simulink model "Modelado_Dron_cuadricoptero_v3"  (R2023a)
settings: Solver=VariableStepAuto  StartTime=0.0  StopTime=10  RelTol=1e-3
libraries: slpidlib x3, sim3dlib x1, uavsim3dlib x1
settings Model: Creator=enzog  LastModifiedBy=enzog

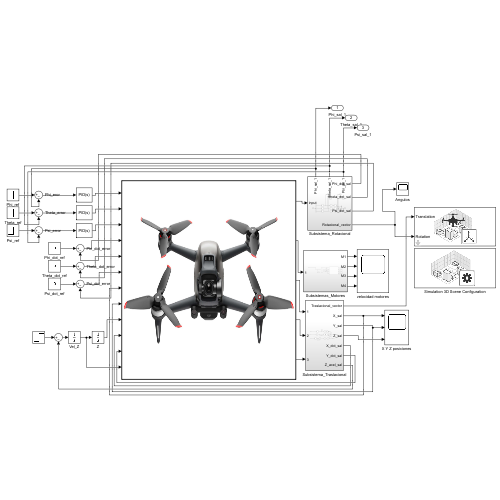
[thumbnail: Simulink's stored preview of the top-level diagram]
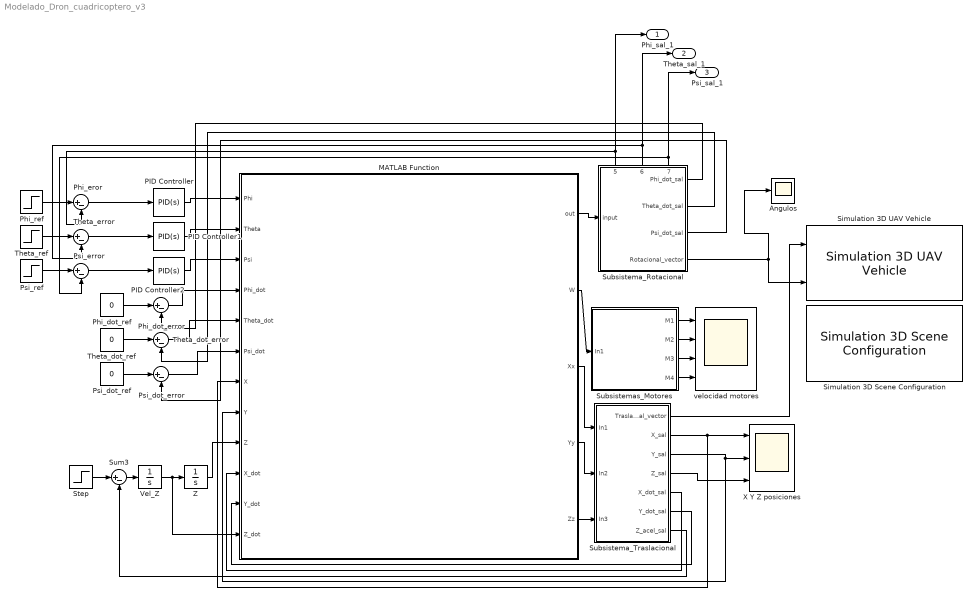
== system Modelado_Dron_cuadricoptero_v3 ==
  Angulos : Scope
  MATLAB Function : MATLAB Function  TreatAsAtomicUnit=on
  PID Controller : slpidlib/PID Controller  Controller=PID  Form=Parallel  TimeDomain=Continuous-time  UseExternalTs=off  SampleTime=-1  IntegratorMethod=Forward Euler  FilterMethod=Forward Euler  ControllerParametersSource=internal  P=150  I=700  UseKiTs=off  D=57  N=100  UseFilter=on  TunerSelectOption=Transfer Function Based (PID Tuner App)  InitialConditionSource=internal  InitialConditionForIntegrator=0  InitialConditionForFilter=0  DifferentiatorICPrevScaledInput=0  ExternalReset=none  TrackingMode=off  Kt=1  LimitOutput=off  SatLimitsSource=internal  UpperSaturationLimit=inf  LowerSaturationLimit=-inf  LinearizeAsGain=on  AntiWindupMode=none  Kb=1  LimitIntegrator=off  UpperIntegratorSaturationLimit=inf  LowerIntegratorSaturationLimit=-inf  POutMin=[]  POutMax=[]  IOutMin=[]  IOutMax=[]  DOutMin=[]  DOutMax=[]  NOutMin=[]  NOutMax=[]  SumOutMin=[]  SumOutMax=[]  SaturationOutMin=[]  SaturationOutMax=[]  PParamMin=[]  PParamMax=[]  IParamMin=[]  IParamMax=[]  DParamMin=[]  DParamMax=[]  NParamMin=[]  NParamMax=[]  KbParamMin=[]  KbParamMax=[]  KtParamMin=[]  KtParamMax=[]  KbOutMin=[]  KbOutMax=[]  KtOutMin=[]  KtOutMax=[]  IntegratorOutMin=[]  IntegratorOutMax=[]  FilterOutMin=[]  FilterOutMax=[]  SumI1OutMin=[]  SumI1OutMax=[]  SumI2OutMin=[]  SumI2OutMax=[]  SumI3OutMin=[]  SumI3OutMax=[]  SumI4OutMin=[]  SumI4OutMax=[]  SumDOutMin=[]  SumDOutMax=[]  DifferentiatorOutMin=[]  DifferentiatorOutMax=[]  FilterDiffOutCoefMin=[]  FilterDiffOutCoefMax=[]  ReciprocalOutMin=[]  ReciprocalOutMax=[]  SumDenOutMin=[]  SumDenOutMax=[]  SumNumOutMin=[]  SumNumOutMax=[]  DivideOutMin=[]  DivideOutMax=[]  UdiffTsProdOutMin=[]  UdiffTsProdOutMax=[]  NTsProdOutMin=[]  NTsProdOutMax=[]  UintegralTsProdOutMin=[]  UintegralTsProdOutMax=[]  UngainTsProdOutMin=[]  UngainTsProdOutMax=[]  ClampingZeroOutDataTypeStr=Inherit: Inherit via back propagation  ClampingZeroOutMin=[]  ClampingZeroOutMax=[]  FilterDenConstantOutDataTypeStr=Inherit: Inherit via back propagation  FilterDenConstantOutMin=[]  FilterDenConstantOutMax=[]  PCopyOutDataTypeStr=Inherit: Inherit via back propagation  PCopyOutMin=[]  PCopyOutMax=[]  NCopyOutDataTypeStr=Inherit: Inherit via back propagation  NCopyOutMin=[]  NCopyOutMax=[]  IntegratorContinuousStateAttributes=''  IntegratorStateMustResolveToSignalObject=off  IntegratorRTWStateStorageClass=Auto  FilterContinuousStateAttributes=''  FilterStateMustResolveToSignalObject=off  FilterRTWStateStorageClass=Auto  ParallelPVariant=InternalParameters  IdealPVariant=Disabled  IVariant=InternalParameters  DVariant=InternalParameters  IntegratorVariant=Continuous  SatVariant=Disabled  AWVariant=Passthrough  PCopyVariant=Disabled  TRVariant=Disabled  FdbkBlocksVariant=Forward  IdealPFdbkVariant=Disabled  SatFdbkVariant=Disabled  DerivativeFilterVariant=ContFilter  NVariant=InternalParameters  NCopyVariant=Disabled  FilterICVariant=InternalICsFilter  IntegratorICVariant=InternalICs  ExternalResetVariant=Disabled  TRSumVariant=Passthrough  SumFdbkVariant=Disabled  SumVariant=Sum_PID  TsampFilterVariant=InternalTs  TsampNgainVariant=Passthrough  TsampIntegralVariant=Disabled_SignalSpec  ExternalSaturationOutDataTypeStr=Inherit: Same as second input
  PID Controller1 : slpidlib/PID Controller  Controller=PID  Form=Parallel  TimeDomain=Continuous-time  UseExternalTs=off  SampleTime=-1  IntegratorMethod=Forward Euler  FilterMethod=Forward Euler  ControllerParametersSource=internal  P=400  I=8.5  UseKiTs=off  D=25  N=100  UseFilter=on  TunerSelectOption=Transfer Function Based (PID Tuner App)  InitialConditionSource=internal  InitialConditionForIntegrator=0  InitialConditionForFilter=0  DifferentiatorICPrevScaledInput=0  ExternalReset=none  TrackingMode=off  Kt=1  LimitOutput=off  SatLimitsSource=internal  UpperSaturationLimit=inf  LowerSaturationLimit=-inf  LinearizeAsGain=on  AntiWindupMode=none  Kb=1  LimitIntegrator=off  UpperIntegratorSaturationLimit=inf  LowerIntegratorSaturationLimit=-inf  POutMin=[]  POutMax=[]  IOutMin=[]  IOutMax=[]  DOutMin=[]  DOutMax=[]  NOutMin=[]  NOutMax=[]  SumOutMin=[]  SumOutMax=[]  SaturationOutMin=[]  SaturationOutMax=[]  PParamMin=[]  PParamMax=[]  IParamMin=[]  IParamMax=[]  DParamMin=[]  DParamMax=[]  NParamMin=[]  NParamMax=[]  KbParamMin=[]  KbParamMax=[]  KtParamMin=[]  KtParamMax=[]  KbOutMin=[]  KbOutMax=[]  KtOutMin=[]  KtOutMax=[]  IntegratorOutMin=[]  IntegratorOutMax=[]  FilterOutMin=[]  FilterOutMax=[]  SumI1OutMin=[]  SumI1OutMax=[]  SumI2OutMin=[]  SumI2OutMax=[]  SumI3OutMin=[]  SumI3OutMax=[]  SumI4OutMin=[]  SumI4OutMax=[]  SumDOutMin=[]  SumDOutMax=[]  DifferentiatorOutMin=[]  DifferentiatorOutMax=[]  FilterDiffOutCoefMin=[]  FilterDiffOutCoefMax=[]  ReciprocalOutMin=[]  ReciprocalOutMax=[]  SumDenOutMin=[]  SumDenOutMax=[]  SumNumOutMin=[]  SumNumOutMax=[]  DivideOutMin=[]  DivideOutMax=[]  UdiffTsProdOutMin=[]  UdiffTsProdOutMax=[]  NTsProdOutMin=[]  NTsProdOutMax=[]  UintegralTsProdOutMin=[]  UintegralTsProdOutMax=[]  UngainTsProdOutMin=[]  UngainTsProdOutMax=[]  ClampingZeroOutDataTypeStr=Inherit: Inherit via back propagation  ClampingZeroOutMin=[]  ClampingZeroOutMax=[]  FilterDenConstantOutDataTypeStr=Inherit: Inherit via back propagation  FilterDenConstantOutMin=[]  FilterDenConstantOutMax=[]  PCopyOutDataTypeStr=Inherit: Inherit via back propagation  PCopyOutMin=[]  PCopyOutMax=[]  NCopyOutDataTypeStr=Inherit: Inherit via back propagation  NCopyOutMin=[]  NCopyOutMax=[]  IntegratorContinuousStateAttributes=''  IntegratorStateMustResolveToSignalObject=off  IntegratorRTWStateStorageClass=Auto  FilterContinuousStateAttributes=''  FilterStateMustResolveToSignalObject=off  FilterRTWStateStorageClass=Auto  ParallelPVariant=InternalParameters  IdealPVariant=Disabled  IVariant=InternalParameters  DVariant=InternalParameters  IntegratorVariant=Continuous  SatVariant=Disabled  AWVariant=Passthrough  PCopyVariant=Disabled  TRVariant=Disabled  FdbkBlocksVariant=Forward  IdealPFdbkVariant=Disabled  SatFdbkVariant=Disabled  DerivativeFilterVariant=ContFilter  NVariant=InternalParameters  NCopyVariant=Disabled  FilterICVariant=InternalICsFilter  IntegratorICVariant=InternalICs  ExternalResetVariant=Disabled  TRSumVariant=Passthrough  SumFdbkVariant=Disabled  SumVariant=Sum_PID  TsampFilterVariant=InternalTs  TsampNgainVariant=Passthrough  TsampIntegralVariant=Disabled_SignalSpec  ExternalSaturationOutDataTypeStr=Inherit: Same as second input
  PID Controller2 : slpidlib/PID Controller  Controller=PID  Form=Parallel  TimeDomain=Continuous-time  UseExternalTs=off  SampleTime=-1  IntegratorMethod=Forward Euler  FilterMethod=Forward Euler  ControllerParametersSource=internal  P=50  I=5.5  UseKiTs=off  D=10  N=100  UseFilter=on  TunerSelectOption=Transfer Function Based (PID Tuner App)  InitialConditionSource=internal  InitialConditionForIntegrator=0  InitialConditionForFilter=0  DifferentiatorICPrevScaledInput=0  ExternalReset=none  TrackingMode=off  Kt=1  LimitOutput=off  SatLimitsSource=internal  UpperSaturationLimit=inf  LowerSaturationLimit=-inf  LinearizeAsGain=on  AntiWindupMode=none  Kb=1  LimitIntegrator=off  UpperIntegratorSaturationLimit=inf  LowerIntegratorSaturationLimit=-inf  POutMin=[]  POutMax=[]  IOutMin=[]  IOutMax=[]  DOutMin=[]  DOutMax=[]  NOutMin=[]  NOutMax=[]  SumOutMin=[]  SumOutMax=[]  SaturationOutMin=[]  SaturationOutMax=[]  PParamMin=[]  PParamMax=[]  IParamMin=[]  IParamMax=[]  DParamMin=[]  DParamMax=[]  NParamMin=[]  NParamMax=[]  KbParamMin=[]  KbParamMax=[]  KtParamMin=[]  KtParamMax=[]  KbOutMin=[]  KbOutMax=[]  KtOutMin=[]  KtOutMax=[]  IntegratorOutMin=[]  IntegratorOutMax=[]  FilterOutMin=[]  FilterOutMax=[]  SumI1OutMin=[]  SumI1OutMax=[]  SumI2OutMin=[]  SumI2OutMax=[]  SumI3OutMin=[]  SumI3OutMax=[]  SumI4OutMin=[]  SumI4OutMax=[]  SumDOutMin=[]  SumDOutMax=[]  DifferentiatorOutMin=[]  DifferentiatorOutMax=[]  FilterDiffOutCoefMin=[]  FilterDiffOutCoefMax=[]  ReciprocalOutMin=[]  ReciprocalOutMax=[]  SumDenOutMin=[]  SumDenOutMax=[]  SumNumOutMin=[]  SumNumOutMax=[]  DivideOutMin=[]  DivideOutMax=[]  UdiffTsProdOutMin=[]  UdiffTsProdOutMax=[]  NTsProdOutMin=[]  NTsProdOutMax=[]  UintegralTsProdOutMin=[]  UintegralTsProdOutMax=[]  UngainTsProdOutMin=[]  UngainTsProdOutMax=[]  ClampingZeroOutDataTypeStr=Inherit: Inherit via back propagation  ClampingZeroOutMin=[]  ClampingZeroOutMax=[]  FilterDenConstantOutDataTypeStr=Inherit: Inherit via back propagation  FilterDenConstantOutMin=[]  FilterDenConstantOutMax=[]  PCopyOutDataTypeStr=Inherit: Inherit via back propagation  PCopyOutMin=[]  PCopyOutMax=[]  NCopyOutDataTypeStr=Inherit: Inherit via back propagation  NCopyOutMin=[]  NCopyOutMax=[]  IntegratorContinuousStateAttributes=''  IntegratorStateMustResolveToSignalObject=off  IntegratorRTWStateStorageClass=Auto  FilterContinuousStateAttributes=''  FilterStateMustResolveToSignalObject=off  FilterRTWStateStorageClass=Auto  ParallelPVariant=InternalParameters  IdealPVariant=Disabled  IVariant=InternalParameters  DVariant=InternalParameters  IntegratorVariant=Continuous  SatVariant=Disabled  AWVariant=Passthrough  PCopyVariant=Disabled  TRVariant=Disabled  FdbkBlocksVariant=Forward  IdealPFdbkVariant=Disabled  SatFdbkVariant=Disabled  DerivativeFilterVariant=ContFilter  NVariant=InternalParameters  NCopyVariant=Disabled  FilterICVariant=InternalICsFilter  IntegratorICVariant=InternalICs  ExternalResetVariant=Disabled  TRSumVariant=Passthrough  SumFdbkVariant=Disabled  SumVariant=Sum_PID  TsampFilterVariant=InternalTs  TsampNgainVariant=Passthrough  TsampIntegralVariant=Disabled_SignalSpec  ExternalSaturationOutDataTypeStr=Inherit: Same as second input
  Phi_dot_error : Sum  Inputs=|+-
  Phi_dot_ref : Constant  Value=0
  Phi_eror : Sum  Inputs=|+-
  Phi_ref : Step  Time=4  After=0.3  SampleTime=0
  Psi_dot_error : Sum  Inputs=|+-
  Psi_dot_ref : Constant  Value=0
  Psi_error : Sum  Inputs=|+-
  Psi_ref : Step  Time=4  After=0.2  SampleTime=0
  Simulation 3D Scene Configuration : sim3dlib/Simulation 3D Scene Configuration  Priority=0  ProjectFormat=Default Scenes  SceneDesc=US city block  ProjectName=C:\Program Files\MATLAB\R2023a\toolbox\shared\sim3d_projects\automotive_project\UE4\WindowsNoEditor\VehicleSimulation.exe  ScenePath=/Game/Maps/USCityBlock  EnableOpenDRIVE=off  vehTagList={'Scene Origin';'SimulinkVehicle1'}  vehTag=SimulinkVehicle1  OpVisEn=off  Ts=1/60  EnableWindow=on  EnableRemoteAccess=off  EnableWeather=off  SunAltitude=40.0  SunAzimuth=90  clouds=10  wind=1  fog=0  rain=0  EnableGeospatial=off  OriginHeight=200  OriginLatitude=40.744652  OriginLongitude=-73.988864  MapStyle=Aerial  AdditionalAssetIDs=[]  UseAdvancedSunSky=off  SolarTime=11  TimeZone=-5  Day=21  Month=9  Year=2022  UseDaylightSavingTime=on  DSTStartDay=10  DSTStartMonth=3  DSTEndDay=3  DSTEndMonth=11  DSTSwitchHour=2  sensorTag=MainCamera1  sensorId=1  sensorName=MainCamera1  mountLoc=Origin  offsetFlag=off  tmountOffset=[0, 0, 0]  rmountOffset=[0, 0, 0]  HorizontalResolution=1280  VerticalResolution=720  HorizontalFOV=60  mountPoint=[0 0 0]  mountOrientation=[0 0 0]  aMode=4  ID=1  GeoTrigger=Inactive
      settings: LibrarySourceBlock=uavsim3dlib/Simulation 3D Scene Configuration
  Simulation 3D UAV Vehicle : uavsim3dlib/Simulation 3D UAV Vehicle  Priority=-1  Mesh=Quadrotor  MeshPath=/MathWorksUAVContent/UAVs/HexaRotorUAV/HexaRotor.HexaRotor  Color=Black  ActorName=SimulinkVehicle1  UseGlobalFrame=off  InitialTranslation=[0 0 0]  InitialRotation=[0 0 0]  InitialTranslationGlobal=[0 0 0]  InitialGeoOrigin=[0 0 0]  InitialRotationGlobal=[0 0 0]  SampleTime=0.01  ActorType=SimulinkVehicle  ID=1  aMode=4  ActorTag=SimulinkVehicle1
  Step : Step  Time=0  After=0.5  SampleTime=0
  Subsistema_Rotacional : Subsystem
      settings: PortSchema="{\"entries\":[{\"content\":{\"sides\":[{\"content\":{\"connectorIds\":[\"In1\"]},\"type\":\"ConnectorPlacement.EquallySpacedRectSide\",\"uuid\":\"c0422ed6-2472-4d81-95b6-acc9af27e97c\"},{\"content\":{\"connectorIds\":[\"Out1\",\"Out2\",\"Out3\",\"Out4\"],\"side\":\"RIGHT\"},\"type\":\"ConnectorPlacement.EquallySpacedRectSide\",\"uuid\":\"ba880dcb-bcf8-4901-b49d-ec4e29830d60\"},{\"content\":{\"connectorIds\":[\"Out5\",\"Out6\",\"Out7\"],\"side\":\"TOP\"},\"type\":\"ConnectorPlacement.EquallySpacedRectSide\",\"uuid\":\"6a94730f-a39a-4262-8327-0681f89bc1da\"}]},\"type\":\"ConnectorPlacement.EquallySpacedConnector\",\"uuid\":\"cda1860d-6ac2-4e1f-973b-4a8b9abeda55\"}],\"packageUris\":[\"http://schema.mathworks.com/mf0/Connector/R2020b\"],\"version\":\"1.0\"}"
  Subsistema_Traslacional : Subsystem
  Subsistemas_Motores : Subsystem
  Sum3 : Sum  Inputs=|+-
  Theta_dot_error : Sum  Inputs=|+-
  Theta_dot_ref : Constant  Value=0
  Theta_error : Sum  Inputs=|+-
  Theta_ref : Step  Time=4  After=-0.45  SampleTime=0
  Vel_Z : Integrator
  X Y Z posiciones : Scope  NumInputPorts=3
  Z : Integrator
  velocidad motores : Scope  NumInputPorts=4
  Phi_sal_1 : Outport
  Theta_sal_1 : Outport  Port=2
  Psi_sal_1 : Outport  Port=3
  wires:
  MATLAB Function/2(W) -> Subsistemas_Motores/1(In1)
  Subsistemas_Motores/1(M1) -> velocidad motores/1
  Subsistemas_Motores/2(M2) -> velocidad motores/2
  Subsistemas_Motores/3(M3) -> velocidad motores/3
  Subsistemas_Motores/4(M4) -> velocidad motores/4
  Subsistema_Rotacional/1(Phi_dot_sal) -> Phi_dot_error/2
  Subsistema_Rotacional/2(Theta_dot_sal) -> Theta_dot_error/2
  Subsistema_Rotacional/3(Psi_dot_sal) -> Psi_dot_error/2
  MATLAB Function/1(out) -> Subsistema_Rotacional/1(input)
  MATLAB Function/3(Xx) -> Subsistema_Traslacional/1(In1)
  MATLAB Function/4(Yy) -> Subsistema_Traslacional/2(In2)
  MATLAB Function/5(Zz) -> Subsistema_Traslacional/3(In3)
  Subsistema_Traslacional/2(X_sal) -> MATLAB Function/7(X), X Y Z posiciones/1
  Subsistema_Traslacional/7(Z_acel_sal) -> Sum3/2
  Subsistema_Traslacional/5(X_dot_sal) -> MATLAB Function/10(X_dot)
  Subsistema_Traslacional/6(Y_dot_sal) -> MATLAB Function/11(Y_dot)
  Subsistema_Traslacional/4(Z_sal) -> X Y Z posiciones/3
  Subsistema_Traslacional/3(Y_sal) -> MATLAB Function/8(Y), X Y Z posiciones/2
  Subsistema_Rotacional/4(Rotacional_vector) -> Angulos/1, Simulation 3D UAV Vehicle/2
  Subsistema_Rotacional/5(Phi_sal_1) -> Phi_sal_1/1, Phi_eror/2
  Subsistema_Rotacional/7(Psi_sal_1) -> Psi_sal_1/1, Psi_error/2
  Phi_dot_ref/1 -> Phi_dot_error/1
  Theta_dot_ref/1 -> Theta_dot_error/1
  Psi_dot_ref/1 -> Psi_dot_error/1
  Phi_dot_error/1 -> MATLAB Function/4(Phi_dot)
  Theta_dot_error/1 -> MATLAB Function/5(Theta_dot)
  Psi_dot_error/1 -> MATLAB Function/6(Psi_dot)
  Subsistema_Traslacional/1(Traslacional_vector) -> Simulation 3D UAV Vehicle/1
  Step/1 -> Sum3/1
  Phi_eror/1 -> PID Controller/1
  PID Controller/1 -> MATLAB Function/1(Phi)
  PID Controller1/1 -> MATLAB Function/2(Theta)
  Theta_error/1 -> PID Controller1/1
  PID Controller2/1 -> MATLAB Function/3(Psi)
  Psi_error/1 -> PID Controller2/1
  Sum3/1 -> Vel_Z/1
  Z/1 -> MATLAB Function/9(Z)
  Vel_Z/1 -> MATLAB Function/12(Z_dot), Z/1
  Theta_ref/1 -> Theta_error/1
  Phi_ref/1 -> Phi_eror/1
  Psi_ref/1 -> Psi_error/1
  Subsistema_Rotacional/6(Theta_sal_1) -> Theta_sal_1/1, Theta_error/2

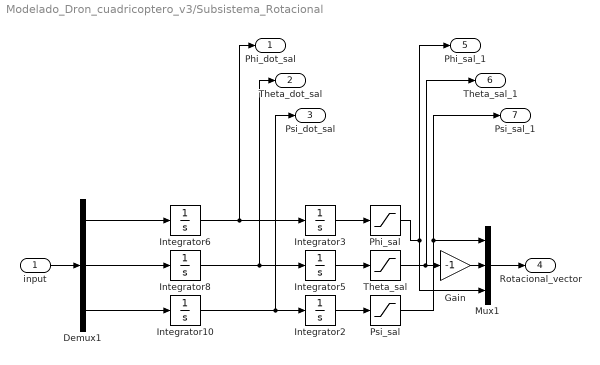
== system Modelado_Dron_cuadricoptero_v3/Subsistema_Rotacional ==
  input : Inport
  Demux1 : Demux  Outputs=3
  Gain : Gain  Gain=-1
  Integrator{2..3,5..6,8,10} (6 alike) : Integrator
  Mux1 : Mux  Inputs=3
  Phi_sal : Saturate  UpperLimit=10  LowerLimit=-10
  Psi_sal : Saturate  UpperLimit=10  LowerLimit=-10
  Theta_sal : Saturate  UpperLimit=10  LowerLimit=-10
  Phi_dot_sal : Outport
  Theta_dot_sal : Outport  Port=2
  Psi_dot_sal : Outport  Port=3
  Rotacional_vector : Outport  Port=4
  Phi_sal_1 : Outport  Port=5
  Theta_sal_1 : Outport  Port=6
  Psi_sal_1 : Outport  Port=7
  wires:
  Demux1/1 -> Integrator6/1
  Demux1/3 -> Integrator10/1
  Integrator8/1 -> Theta_dot_sal/1, Integrator5/1
  Demux1/2 -> Integrator8/1
  Mux1/1 -> Rotacional_vector/1
  Integrator10/1 -> Psi_dot_sal/1, Integrator2/1
  Integrator6/1 -> Integrator3/1, Phi_dot_sal/1
  input/1 -> Demux1/1
  Integrator3/1 -> Phi_sal/1
  Integrator2/1 -> Psi_sal/1
  Integrator5/1 -> Theta_sal/1
  Phi_sal/1 -> Mux1/3, Phi_sal_1/1
  Theta_sal/1 -> Gain/1, Theta_sal_1/1
  Psi_sal/1 -> Mux1/1, Psi_sal_1/1
  Gain/1 -> Mux1/2

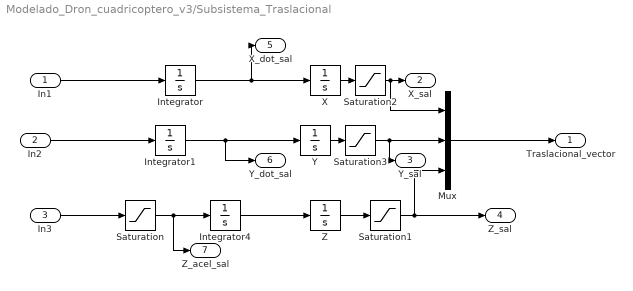
== system Modelado_Dron_cuadricoptero_v3/Subsistema_Traslacional ==
  In1 : Inport
  In2 : Inport  Port=2
  In3 : Inport  Port=3
  Integrator : Integrator
  Integrator1 : Integrator
  Integrator4 : Integrator
  Mux : Mux  Inputs=3
  Saturation : Saturate  UpperLimit=2  LowerLimit=-2
  Saturation1 : Saturate  UpperLimit=80  LowerLimit=-80
  Saturation2 : Saturate  UpperLimit=80  LowerLimit=-80
  Saturation3 : Saturate  UpperLimit=80  LowerLimit=-80
  X : Integrator
  Y : Integrator
  Z : Integrator
  Traslacional_vector : Outport
  X_sal : Outport  Port=2
  Y_sal : Outport  Port=3
  Z_sal : Outport  Port=4
  X_dot_sal : Outport  Port=5
  Y_dot_sal : Outport  Port=6
  Z_acel_sal : Outport  Port=7
  wires:
  Integrator/1 -> X/1, X_dot_sal/1
  X/1 -> Saturation2/1
  Saturation/1 -> Z_acel_sal/1, Integrator4/1
  Integrator4/1 -> Z/1
  Integrator1/1 -> Y/1, Y_dot_sal/1
  In3/1 -> Saturation/1
  Z/1 -> Saturation1/1
  Mux/1 -> Traslacional_vector/1
  In2/1 -> Integrator1/1
  In1/1 -> Integrator/1
  Y/1 -> Saturation3/1
  Saturation3/1 -> Y_sal/1, Mux/2
  Saturation1/1 -> Z_sal/1, Mux/3
  Saturation2/1 -> X_sal/1, Mux/1

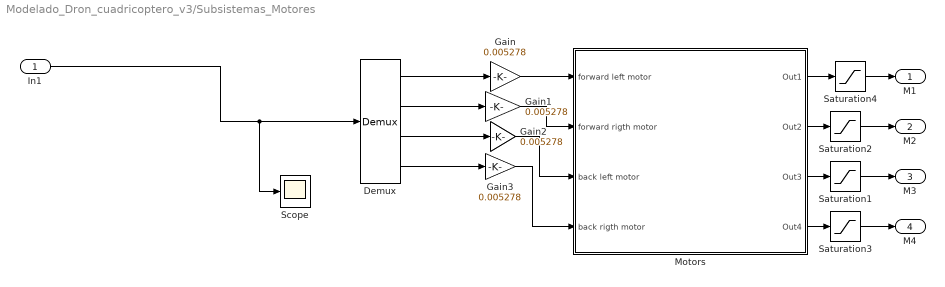
== system Modelado_Dron_cuadricoptero_v3/Subsistemas_Motores ==
  In1 : Inport
  Demux : Demux
      settings: DisplayOption=none
  Gain{,1..3} (4 alike) : Gain  Gain=0.005278
  Motors : Subsystem
  Saturation{1..4} (4 alike) : Saturate  UpperLimit=2103  LowerLimit=0
  Scope : Scope
  M1 : Outport
  M2 : Outport  Port=2
  M3 : Outport  Port=3
  M4 : Outport  Port=4
  wires:
  Motors/1(Out1) -> Saturation4/1
  Gain1/1 -> Motors/2(forward rigth motor)
  Saturation2/1 -> M2/1
  Saturation1/1 -> M3/1
  Demux/2 -> Gain1/1
  Demux/1 -> Gain/1
  Gain/1 -> Motors/1(forward left motor)
  Motors/4(Out4) -> Saturation3/1
  Gain3/1 -> Motors/4(back rigth motor)
  Saturation4/1 -> M1/1
  Saturation3/1 -> M4/1
  Gain2/1 -> Motors/3(back left motor)
  Demux/4 -> Gain3/1
  Motors/3(Out3) -> Saturation1/1
  Demux/3 -> Gain2/1
  Motors/2(Out2) -> Saturation2/1
  In1/1 -> Scope/1, Demux/1

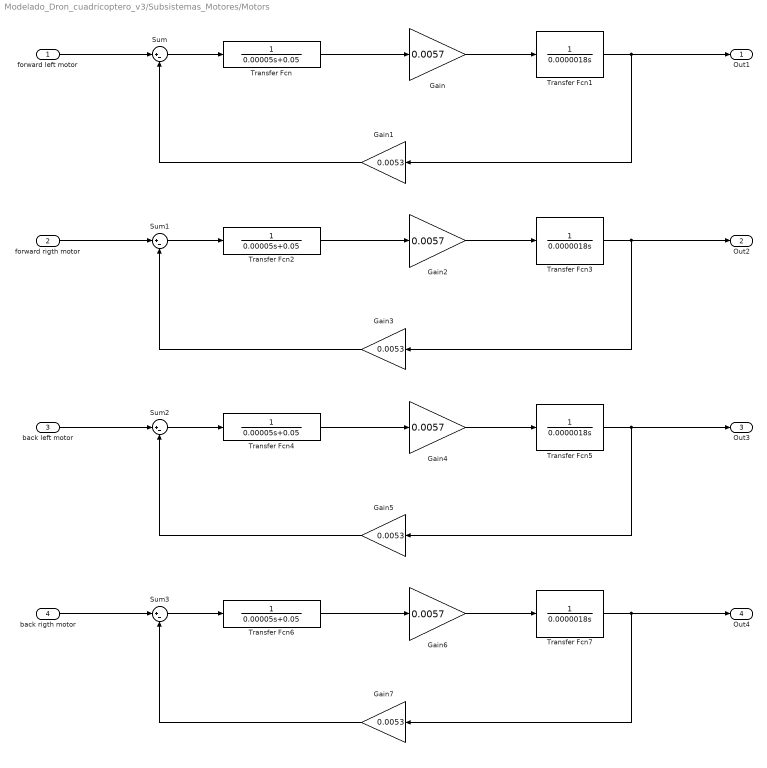
== system Modelado_Dron_cuadricoptero_v3/Subsistemas_Motores/Motors ==
  forward left motor : Inport
  forward rigth motor : Inport  Port=2
  back left motor : Inport  Port=3
  back rigth motor : Inport  Port=4
  Gain{,2,4,6} (4 alike) : Gain  Gain=0.0057
  Gain{1,3,5,7} (4 alike) : Gain  Gain=0.0053
  Sum{,1..3} (4 alike) : Sum  Inputs=|+-
  Transfer Fcn{,2,4,6} (4 alike) : TransferFcn  Denominator=[0.00005 0.05]
  Transfer Fcn{1,3,5,7} (4 alike) : TransferFcn  Denominator=[0.0000018 0]
  Out1 : Outport
  Out2 : Outport  Port=2
  Out3 : Outport  Port=3
  Out4 : Outport  Port=4
  wires:
  Gain/1 -> Transfer Fcn1/1
  Transfer Fcn/1 -> Gain/1
  Gain1/1 -> Sum/2
  Transfer Fcn1/1 -> Out1/1, Gain1/1
  Sum/1 -> Transfer Fcn/1
  Sum1/1 -> Transfer Fcn2/1
  Transfer Fcn3/1 -> Out2/1, Gain3/1
  Gain3/1 -> Sum1/2
  Transfer Fcn2/1 -> Gain2/1
  Gain2/1 -> Transfer Fcn3/1
  Sum2/1 -> Transfer Fcn4/1
  Transfer Fcn5/1 -> Out3/1, Gain5/1
  Gain5/1 -> Sum2/2
  Transfer Fcn4/1 -> Gain4/1
  Gain4/1 -> Transfer Fcn5/1
  Sum3/1 -> Transfer Fcn6/1
  Transfer Fcn7/1 -> Out4/1, Gain7/1
  Gain7/1 -> Sum3/2
  Transfer Fcn6/1 -> Gain6/1
  Gain6/1 -> Transfer Fcn7/1
  back rigth motor/1 -> Sum3/1
  back left motor/1 -> Sum2/1
  forward rigth motor/1 -> Sum1/1
  forward left motor/1 -> Sum/1

== matlab function Modelado_Dron_cuadricoptero_v3/MATLAB Function ==
  data: Phi input size=1; out output size=[3,1]; Theta input size=1; Psi input size=1; Phi_dot input size=1; Theta_dot input size=1; Psi_dot input size=1; X input size=1; Y input size=1; Z input size=1; X_dot input size=1; Y_dot input size=1; Z_dot input size=1; W output size=[4,1]; Xx output size=1; Yy output size=1; Zz output size=1
function [out,W,Xx,Yy,Zz]= DronCuadricopteroV2(Phi,Theta,Psi,Phi_dot,Theta_dot,Psi_dot,X,Y,Z,X_dot,Y_dot,Z_dot)

%--------------------------------PARAMETROS (SI)-------------------------

Ix = 0.00298; % Kg*m^2
Iy = 0.00298; % Kg*m^2
Iz = 0.006;   % Kg*m^2
M = 0.720;    % kg
l = 0.2;      % m
g = 9.81;     % m/s^2
K = 0.00000273;
b = 0.0000001;
Ax = 0.2;
Ay = 0.2;
Az = 0.2;

%-------------------------------DEF. VAR.LOCALES-------------------------

Phi_local = Phi;
Theta_local = Theta;
Psi_local = Psi;
Phi_dot_local = Phi_dot;
Theta_dot_local = Theta_dot;
Psi_dot_local = Psi_dot;
X_local = X;
Y_local = Y;
Z_local = Z;
X_dot_local = X_dot;
Y_dot_local = Y_dot;
Z_dot_local = Z_dot;

%-------------------------------TORQUES Y VELOCIDADES-------------------

Tau_Phi = Ix*(Phi_dot_local + Phi_local);
Tau_Theta = Iy*(Theta_dot_local + Theta_local);
Tau_Psi = Iz*(Psi_dot_local + Psi_local);

T = (g + Z_dot_local + Z_local)*M;

W = [1 -1 1 1;1 1 -1 1;1 1 1 -1;1 -1 -1 -1]*[T/(0.01);Tau_Theta;Tau_Phi;Tau_Psi]; %se divide para que arranque en 700 


%-------------------------------J y C-----------------------------------

J = zeros(3,3);
C = zeros(3,3);

J(1,1) = Ix;
J(1,2) = 0;
J(1,3) = -Ix*Theta_local;
J(2,1) = 0;
J(2,2) = Iy + Iz*(Phi_local)^2;
J(2,3) = (Iy-Iz)*Phi_local;
J(3,1) = -Ix*Theta_local;
J(3,2) = (Iy-Iz)*Phi_local;
J(3,3) = Ix*(Theta_local)^2 + Iy*(Phi_local)^2 + Iz;

C(1,1) = 0;
C(1,2) = (Iy-Iz)*(Theta_dot_local*Phi_local + Psi_dot_local*(Phi_local)^2) + (Iz-Iy)*Psi_dot_local + Ix*Psi_dot_local;
C(1,3) = (Iz-Iy)*Psi_dot_local*Phi_local;
C(2,1) = (Iz-Iy)*(Theta_dot_local*Phi_local + Psi_dot_local*Phi_local) + (Iy-Iz)*Psi_dot_local + Ix*Psi_dot_local;
C(2,2) = (Iz-Iy)*Phi_dot_local*Phi_local;
C(2,3) = -Ix*Psi_dot_local*Theta_local + Iy*Psi_dot_local*(Phi_local)^2*Theta_local + Iz*Psi_dot_local*Theta_local;
C(3,1) = (Iy-Iz)*Psi_dot_local*Phi_local - Ix*Theta_dot_local;
C(3,2) = (Iz-Iy)*(Theta_dot_local*Phi_local*Theta_local + Phi_dot_local*(Phi_local)^2) + (Iy-Iz)*Phi_dot_local + Ix*Psi_dot_local*Theta_local - Iy*Psi_dot_local*(Phi_local)^2*Theta_local - Iz*Psi_dot_local*Theta_local;
C(3,3) = (Iy-Iz)*Phi_dot_local*Phi_local - Iy*Theta_dot_local*(Phi_local)^2*Theta_local - Iz*Theta_dot_local*Theta_local + Ix*Theta_dot_local*Theta_local;

%----------------------------PARTE FINAL--------------------------------

B = [Tau_Phi,Tau_Theta,Tau_Psi]';

N = [Phi_dot_local,Theta_dot_local,Psi_dot_local]';

% W = [W1 W2 W3 W4];

z_ddot = (T/M) - g - (Az/M)*Z_dot_local;
x_ddot = (T/M)*((-Theta_local/10) + (Phi_local/150)*(Psi_local/50)) ;% (Ax/M)*X_dot_local;
y_ddot = (T/M)*((Theta_local/400)*(Psi_local/50) - (Phi_local/10)) ;% (Ay/M)*Y_dot_local;%(-Phi_local + Theta_local*Psi_local)

Xx = x_ddot;
Yy = y_ddot;
Zz = z_ddot;

Hh = inv(J)*(B-C*N);

out = Hh;

end


% W1 = ((T/(4*K) - Tau_Phi/(b) + Tau_Theta/(b) + Tau_Psi/(b))^2)^0.25;
% W2 = ((T/(4*K) + Tau_Phi/(b) + Tau_Theta/(b) - Tau_Psi/(b))^2)^0.25;
% W3 = ((T/(4*K) + Tau_Phi/(b) - Tau_Theta/(b) + Tau_Psi/(b))^2)^0.25;
% W4 = ((T/(4*K) - Tau_Phi/(b) - Tau_Theta/(b) - Tau_Psi/(b))^2)^0.25;

% W1 = (T/(4*K)  + Tau_Theta(2*K*l) + Tau_Psi/(4*b))^2;
% W2 = 0.25*(T/(4*K) - Tau_Theta(2*K*l) + Tau_Psi/(4*b));
% W3 = 0.25*(T/(4*K)  + Tau_Theta(2*K*l) - Tau_Psi/(4*b));
% W4 = 0.25*(T/(4*K)  - Tau_Theta(2*K*l) - Tau_Psi/(4*b));

 % W1 = ((T/(4*K) - 3*Tau_Theta/(K) - 3*Tau_Psi/(2*b))^2)^0.25;
 % W2 = ((T/(4*K) - 3*Tau_Phi/(K) + 3*Tau_Psi/(2*b))^2)^0.25;    %REVEER%
 % W3 = ((T/(4*K) + 3*Tau_Theta/(K) - 3*Tau_Psi/(2*b))^2)^0.25; % original: (T/(4*K) + Tau_Theta/(2*K*l) - Tau_Psi/(4*b))^0.5
 % W4 = ((T/(4*K) + 3*Tau_Phi/(K) + 3*Tau_Psi/(2*b))^2)^0.25;


%Ww = [1 1 1 1 ; -1 1 1 -1 ; 1 1 -1 -1 ; 1 -1 1 -1];

%W = inv(Ww)*[N11;N12;N21;N22];
